simulink model "QPSK_Transmit_v3"  (R2012b)
settings: Solver=FixedStepDiscrete  StartTime=0.0  StopTime=150  FixedStep=1  RelTol=1e-3
libraries: simulink x23, commutil2 x3
settings Model: Creator=Carl  LastModifiedBy=Carl
settings DataIOCC: SignalLogging=off
settings OptimizationCC: BlockReduction=off  ConditionallyExecuteInputs=off  InlineParams=on
settings DebuggingCC: AlgebraicLoopMsg=error
settings HardwareCC: ProdHWDeviceType=ASIC/FPGA->ASIC/FPGA  ProdEqTarget=off

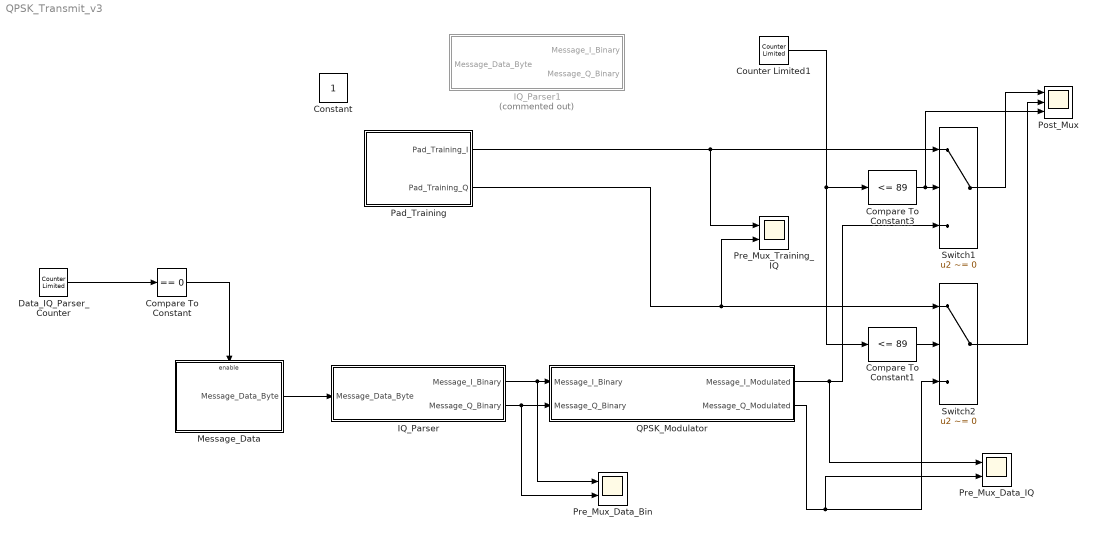
== system QPSK_Transmit_v3 ==
  Compare To Constant1 : simulink/Logic and Bit Operations/Compare To Constant  relop=<=  const=89  OutDataTypeStr=boolean  ZeroCross=off
  Compare To Constant3 : simulink/Logic and Bit Operations/Compare To Constant  relop=<=  const=89  OutDataTypeStr=boolean  ZeroCross=off
  Compare To Constant : simulink/Logic and Bit Operations/Compare To Constant  relop===  const=0  OutDataTypeStr=boolean
  Constant : Constant  OutDataTypeStr=boolean
  Counter Limited1 : simulink/Sources/Counter Limited  uplimit=1023  tsamp=-1
  Data_IQ_Parser_Counter : simulink/Sources/Counter Limited  uplimit=3  tsamp=-1
  IQ_Parser : Subsystem
  IQ_Parser1 : Subsystem  Commented=on
  Message_Data : Subsystem
  Pad_Training : Subsystem
  Post_Mux : Scope  NumInputPorts=3
      settings: YMin=-5~-5~-5  YMax=5~5~5  SaveName=ScopeData2
  Pre_Mux_Data_Bin : Scope  NumInputPorts=2
      settings: YMin=-5~-5  YMax=5~5  SaveName=ScopeData6
  Pre_Mux_Data_IQ : Scope  NumInputPorts=2
      settings: YMin=-5~-5  YMax=5~5  SaveName=ScopeData5
  Pre_Mux_Training_IQ : Scope  NumInputPorts=2
      settings: YMin=-5~-5  YMax=5~5  SaveName=ScopeData4
  QPSK_Modulator : Subsystem
  Switch1 : Switch  Criteria=u2 ~= 0  OutDataTypeStr=int8
  Switch2 : Switch  Criteria=u2 ~= 0  OutDataTypeStr=int8
  wires:
  Compare To Constant3/1 -> Post_Mux/3, Switch1/2
  Counter Limited1/1 -> Compare To Constant1/1, Compare To Constant3/1
  Switch1/1 -> Post_Mux/1
  Pad_Training/1(Pad_Training_I) -> Pre_Mux_Training_IQ/1, Switch1/1
  Compare To Constant1/1 -> Switch2/2
  Switch2/1 -> Post_Mux/2
  Pad_Training/2(Pad_Training_Q) -> Pre_Mux_Training_IQ/2, Switch2/1
  Message_Data/1(Message_Data_Byte) -> IQ_Parser/1(Message_Data_Byte)
  IQ_Parser/1(Message_I_Binary) -> Pre_Mux_Data_Bin/1, QPSK_Modulator/1(Message_I_Binary)
  IQ_Parser/2(Message_Q_Binary) -> Pre_Mux_Data_Bin/2, QPSK_Modulator/2(Message_Q_Binary)
  QPSK_Modulator/1(Message_I_Modulated) -> Pre_Mux_Data_IQ/1, Switch1/3
  QPSK_Modulator/2(Message_Q_Modulated) -> Pre_Mux_Data_IQ/2, Switch2/3
  Data_IQ_Parser_Counter/1 -> Compare To Constant/1
  Compare To Constant/1 -> Message_Data/Enable

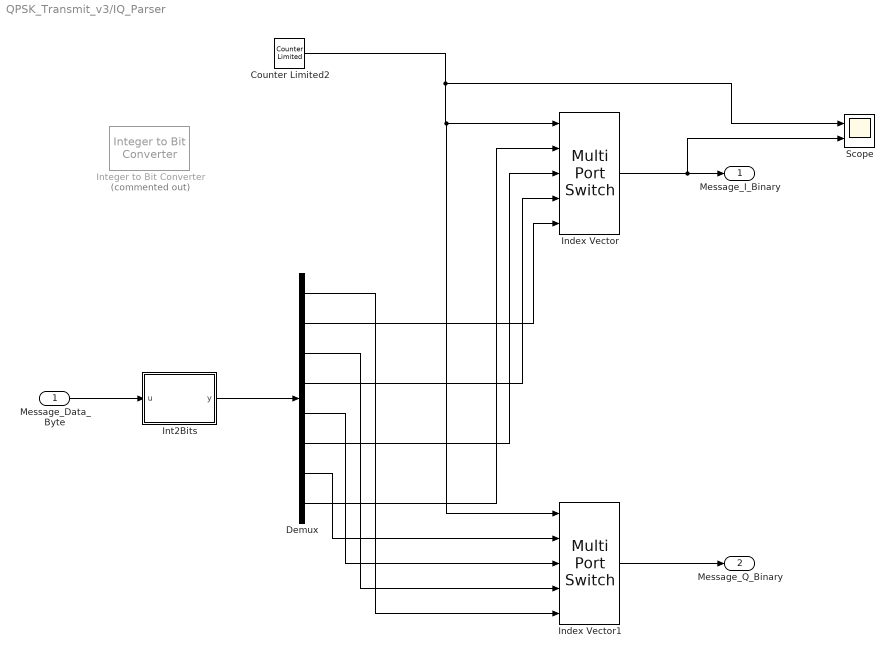
== system QPSK_Transmit_v3/IQ_Parser ==
  Message_Data_Byte : Inport
  Counter Limited2 : simulink/Sources/Counter Limited  uplimit=3  tsamp=-1
  Demux : Demux  Outputs=8
  Index Vector : MultiPortSwitch  DataPortOrder=Zero-based contiguous  Inputs=4  zeroidx=on
  Index Vector1 : MultiPortSwitch  DataPortOrder=Zero-based contiguous  Inputs=4  zeroidx=on
  Int2Bits : MATLAB Function  TreatAsAtomicUnit=on
  Integer to Bit Converter : commutil2/Integer to Bit Converter  Commented=on  nbits=8  signedInputValues=Unsigned  bitOrder=MSB first  outDtype=Inherit via internal rule
  Scope : Scope  NumInputPorts=2
      settings: YMin=-5~-5  YMax=5~5
  Message_I_Binary : Outport
  Message_Q_Binary : Outport  Port=2
  wires:
  Index Vector1/1 -> Message_Q_Binary/1
  Counter Limited2/1 -> Scope/1, Index Vector/1, Index Vector1/1
  Index Vector/1 -> Scope/2, Message_I_Binary/1
  Demux/8 -> Index Vector/2
  Demux/7 -> Index Vector1/2
  Demux/6 -> Index Vector/3
  Demux/5 -> Index Vector1/3
  Demux/4 -> Index Vector/4
  Demux/3 -> Index Vector1/4
  Demux/2 -> Index Vector/5
  Demux/1 -> Index Vector1/5
  Message_Data_Byte/1 -> Int2Bits/1(u)
  Int2Bits/1(y) -> Demux/1

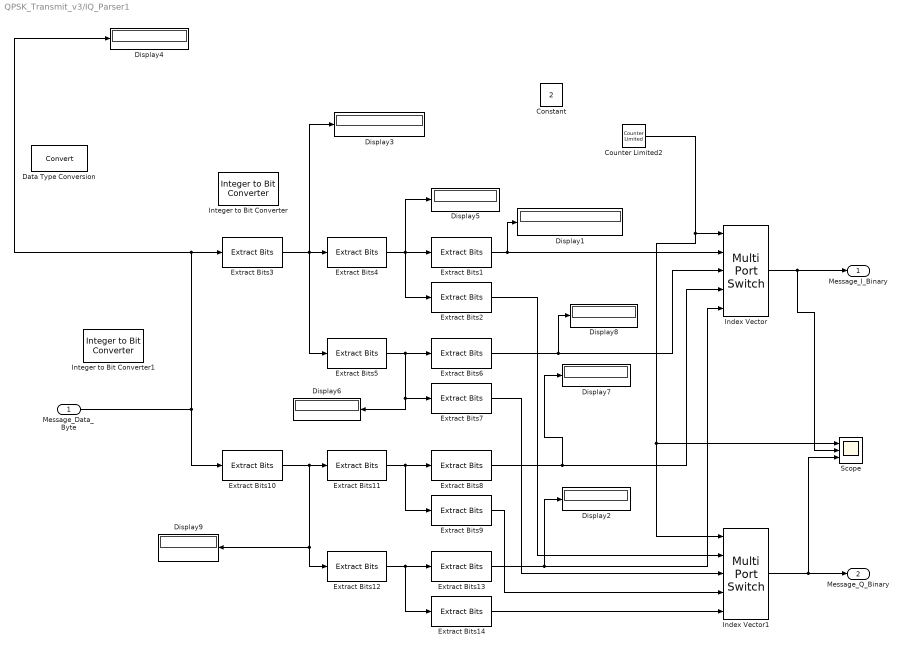
== system QPSK_Transmit_v3/IQ_Parser1 ==
  Message_Data_Byte : Inport
  Constant : Constant  Value=2
  Counter Limited2 : simulink/Sources/Counter Limited  uplimit=3  tsamp=-1
  Data Type Conversion : DataTypeConversion  ConvertRealWorld=Stored Integer (SI)  RndMeth=Nearest
  Display{1..9} (9 alike) : Display
      Display1 settings: Format=binary (Stored Integer)
      Display3 settings: Format=binary (Stored Integer)
      Display4 settings: Format=binary (Stored Integer)
      Display5 settings: Format=binary (Stored Integer)
      Display6 settings: Format=binary (Stored Integer)
      Display8 settings: Format=binary (Stored Integer)
      Display9 settings: Format=binary (Stored Integer)
  Extract Bits1 : simulink/Logic and Bit Operations/Extract Bits  bitsToExtract=Upper half  numBits=1  bitIdxRange=[15]  outScalingMode=Preserve fixed-point scaling
  Extract Bits10 : simulink/Logic and Bit Operations/Extract Bits  bitsToExtract=Lower half  numBits=2  bitIdxRange=[1 3 5 7]  outScalingMode=Preserve fixed-point scaling
  Extract Bits11 : simulink/Logic and Bit Operations/Extract Bits  bitsToExtract=Upper half  numBits=2  bitIdxRange=[0 2 4 6]  outScalingMode=Preserve fixed-point scaling
  Extract Bits12 : simulink/Logic and Bit Operations/Extract Bits  bitsToExtract=Lower half  numBits=2  bitIdxRange=[0 2 4 6]  outScalingMode=Preserve fixed-point scaling
  Extract Bits13 : simulink/Logic and Bit Operations/Extract Bits  bitsToExtract=Upper half  numBits=1  bitIdxRange=[15]  outScalingMode=Preserve fixed-point scaling
  Extract Bits{2,7,9,14} (4 alike) : simulink/Logic and Bit Operations/Extract Bits  bitsToExtract=Lower half  numBits=1  bitIdxRange=[15]  outScalingMode=Preserve fixed-point scaling
  Extract Bits3 : simulink/Logic and Bit Operations/Extract Bits  bitsToExtract=Upper half  numBits=4  bitIdxRange=[0 2 4 6]  outScalingMode=Preserve fixed-point scaling
  Extract Bits4 : simulink/Logic and Bit Operations/Extract Bits  bitsToExtract=Upper half  numBits=2  bitIdxRange=[0 2 4 6]  outScalingMode=Preserve fixed-point scaling
  Extract Bits5 : simulink/Logic and Bit Operations/Extract Bits  bitsToExtract=Lower half  numBits=2  bitIdxRange=[0 2 4 6]  outScalingMode=Preserve fixed-point scaling
  Extract Bits6 : simulink/Logic and Bit Operations/Extract Bits  bitsToExtract=Range starting with most significant bit  numBits=1  bitIdxRange=[15]  outScalingMode=Preserve fixed-point scaling
  Extract Bits8 : simulink/Logic and Bit Operations/Extract Bits  bitsToExtract=Upper half  numBits=1  bitIdxRange=[15]  outScalingMode=Preserve fixed-point scaling
  Index Vector : MultiPortSwitch  DataPortOrder=Zero-based contiguous  Inputs=4  zeroidx=on
  Index Vector1 : MultiPortSwitch  DataPortOrder=Zero-based contiguous  Inputs=4  zeroidx=on
  Integer to Bit Converter : commutil2/Integer to Bit Converter  nbits=8  signedInputValues=Unsigned  bitOrder=MSB first  outDtype=Inherit via internal rule
  Integer to Bit Converter1 : commutil2/Integer to Bit Converter  nbits=8  signedInputValues=Unsigned  bitOrder=MSB first  outDtype=Inherit via internal rule
  Scope : Scope  NumInputPorts=3
      settings: YMin=-5~-5~-5  YMax=5~5~5
  Message_I_Binary : Outport
  Message_Q_Binary : Outport  Port=2
  wires:
  Index Vector1/1 -> Scope/3, Message_Q_Binary/1
  Extract Bits3/1 -> Display3/1, Extract Bits5/1, Extract Bits4/1
  Extract Bits4/1 -> Display5/1, Extract Bits2/1, Extract Bits1/1
  Extract Bits5/1 -> Extract Bits6/1, Display6/1, Extract Bits7/1
  Extract Bits10/1 -> Extract Bits11/1, Extract Bits12/1, Display9/1
  Extract Bits11/1 -> Extract Bits8/1, Extract Bits9/1
  Extract Bits12/1 -> Extract Bits14/1, Extract Bits13/1
  Extract Bits2/1 -> Index Vector1/2
  Extract Bits7/1 -> Index Vector1/3
  Extract Bits8/1 -> Display7/1, Index Vector/4
  Extract Bits9/1 -> Index Vector1/4
  Extract Bits13/1 -> Display2/1, Index Vector/5
  Extract Bits14/1 -> Index Vector1/5
  Index Vector/1 -> Scope/2, Message_I_Binary/1
  Counter Limited2/1 -> Index Vector1/1, Scope/1, Index Vector/1
  Extract Bits1/1 -> Index Vector/2, Display1/1
  Extract Bits6/1 -> Index Vector/3, Display8/1
  Message_Data_Byte/1 -> Extract Bits10/1, Extract Bits3/1, Display4/1

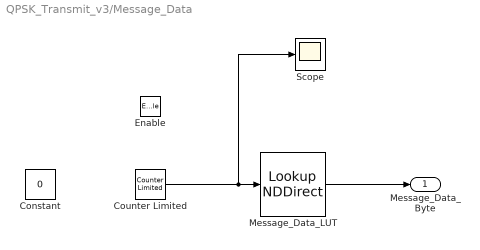
== system QPSK_Transmit_v3/Message_Data ==
  Enable : EnablePort
  Constant : Constant  Value=0
  Counter Limited : simulink/Sources/Counter Limited  uplimit=17  tsamp=-1
  Message_Data_LUT : LookupNDDirect  NumberOfTableDimensions=1  Table="[12        0        0        1        104        101        108        108        111        32        119        111        114        108        100        33        198        228]"  DiagnosticForOutOfRangeInput=Error  TableDataTypeStr=uint8
  Scope : Scope
  Message_Data_Byte : Outport
  wires:
  Message_Data_LUT/1 -> Message_Data_Byte/1
  Counter Limited/1 -> Scope/1, Message_Data_LUT/1

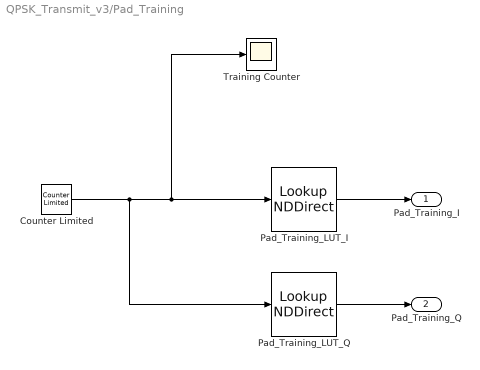
== system QPSK_Transmit_v3/Pad_Training ==
  Counter Limited : simulink/Sources/Counter Limited  uplimit=89  tsamp=-1
  Pad_Training_LUT_I : LookupNDDirect  NumberOfTableDimensions=1  Table=[1,-1,1,-1,1,-1,1,-1,1,-1,1,-1,1,-1,1,-1,1,-1,1,-1,1,-1,1,-1,1,1,1,-1,-1,1,1,-1,-1,1,-1,-1,-1,-1,1,-1,1,1,-1,-1,1,1,1,-1,1,1,1,-1,1,-1,1,1,1,-1,1,1,1,1,-1,1,1,-1,-1,-1,-1,1,1,1,-1,-1,-1,1,1,1,1,-1,1,1,1,1,1,-1,-1,-1,1,1]  DiagnosticForOutOfRangeInput=Error  TableDataTypeStr=int8
  Pad_Training_LUT_Q : LookupNDDirect  NumberOfTableDimensions=1  Table=[1,-1,1,-1,1,-1,1,-1,1,-1,1,-1,1,-1,1,-1,1,-1,1,-1,1,-1,1,-1,1,1,-1,1,1,1,-1,-1,-1,-1,1,1,-1,1,1,-1,-1,-1,1,-1,-1,1,1,1,-1,-1,1,1,1,-1,-1,-1,-1,-1,-1,1,1,-1,1,-1,1,1,-1,-1,1,-1,-1,1,1,-1,-1,-1,-1,-1,1,1,1,1,-1,-1,-1,-1,1,-1,1,-1]  DiagnosticForOutOfRangeInput=Error  TableDataTypeStr=int8
  Training Counter : Scope
      settings: SaveName=ScopeData3
  Pad_Training_I : Outport
  Pad_Training_Q : Outport  Port=2
  wires:
  Pad_Training_LUT_I/1 -> Pad_Training_I/1
  Counter Limited/1 -> Training Counter/1, Pad_Training_LUT_I/1, Pad_Training_LUT_Q/1
  Pad_Training_LUT_Q/1 -> Pad_Training_Q/1

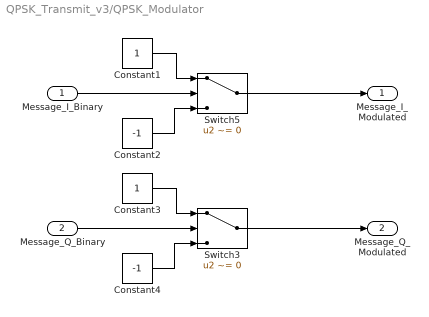
== system QPSK_Transmit_v3/QPSK_Modulator ==
  Message_I_Binary : Inport
  Message_Q_Binary : Inport  Port=2
  Constant1 : Constant  OutDataTypeStr=int8
  Constant2 : Constant  Value=-1  OutDataTypeStr=int8
  Constant3 : Constant  OutDataTypeStr=int8
  Constant4 : Constant  Value=-1  OutDataTypeStr=int8
  Switch3 : Switch  Criteria=u2 ~= 0  RndMeth=Round
  Switch5 : Switch  Criteria=u2 ~= 0  RndMeth=Round
  Message_I_Modulated : Outport
  Message_Q_Modulated : Outport  Port=2
  wires:
  Switch3/1 -> Message_Q_Modulated/1
  Constant4/1 -> Switch3/3
  Constant2/1 -> Switch5/3
  Constant1/1 -> Switch5/1
  Message_Q_Binary/1 -> Switch3/2
  Constant3/1 -> Switch3/1
  Switch5/1 -> Message_I_Modulated/1
  Message_I_Binary/1 -> Switch5/2

== matlab function QPSK_Transmit_v3/IQ_Parser/Int2Bits ==
  data: u input; y output
function y = fcn(u)
% Converts Integer(8bits) to a 1-D array Bits

y = bitget(u, [8:-1:1])';
